simulink model "three"  (R2020b)
settings: Solver=FixedStepAuto  StartTime=0.0  StopTime=0.5  FixedStep=0.00005  RelTol=1e-3
libraries: simulink x3
settings Model: Creator=13228  LastModifiedBy=up!

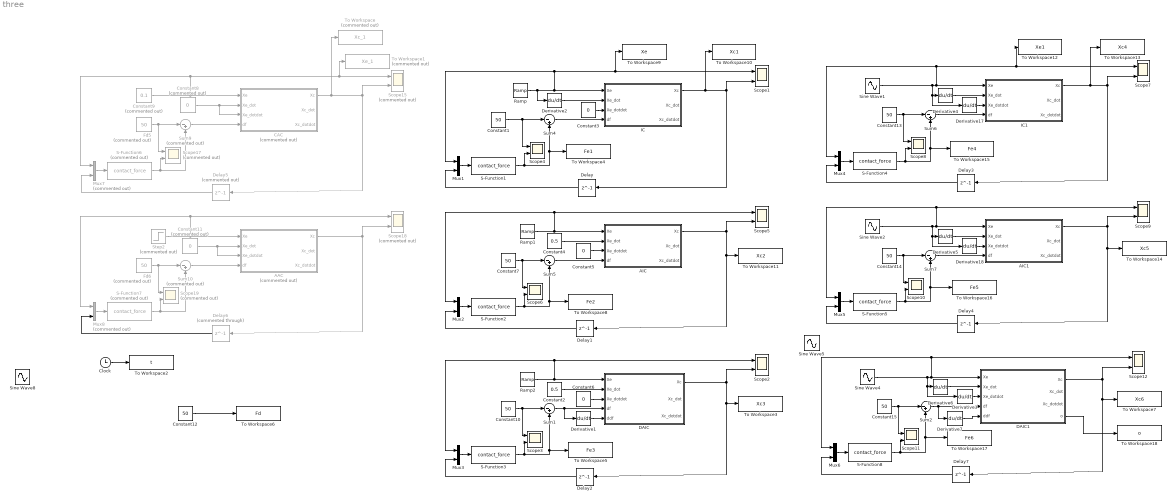
== system three ==
  AAC : MATLAB Function  Commented=on  TreatAsAtomicUnit=on
  AIC : MATLAB Function  TreatAsAtomicUnit=on
  AIC1 : MATLAB Function  TreatAsAtomicUnit=on
  CAC : MATLAB Function  Commented=on  TreatAsAtomicUnit=on
  Clock : Clock
  Constant{1,7,10,13..15} (6 alike) : Constant  Value=50
  Constant11 : Constant  Commented=on  Value=0
  Constant12 : Constant  Value=50  SampleTime=0.1
  Constant2 : Constant  Value=0.5
  Constant3 : Constant  Value=0
  Constant4 : Constant  Value=0.5
  Constant5 : Constant  Value=0
  Constant6 : Constant  Value=0
  Constant8 : Constant  Commented=on  Value=0
  Constant9 : Constant  Commented=on  Value=0.1
  DAIC : MATLAB Function  TreatAsAtomicUnit=on
  DAIC1 : MATLAB Function  TreatAsAtomicUnit=on
  Delay : Delay  DelayLength=1  InitialCondition=-0.002
  Delay1 : Delay  DelayLength=1  InitialCondition=-0.002
  Delay2 : Delay  DelayLength=1  InitialCondition=-0.002
  Delay3 : Delay  DelayLength=1  InitialCondition=0.098
  Delay4 : Delay  DelayLength=1  InitialCondition=0.098
  Delay5 : Delay  Commented=on  DelayLength=1  InitialCondition=0.098
  Delay6 : Delay  Commented=through  DelayLength=1  InitialCondition=0.098
  Delay7 : Delay  DelayLength=1  InitialCondition=0.098
  Derivative{1..7,17..18} (9 alike) : Derivative
  Fd5 : Constant  Commented=on  Value=50
  Fd6 : Constant  Commented=on  Value=50
  IC : MATLAB Function  TreatAsAtomicUnit=on
  IC1 : MATLAB Function  TreatAsAtomicUnit=on
  Mux{1..6} (6 alike) : Mux  Inputs=2
  Mux7 : Mux  Commented=on  Inputs=2
  Mux8 : Mux  Commented=on  Inputs=2
  Ramp : simulink/Sources/Ramp  slope=0.5  start=0.001  InitialOutput=0
  Ramp1 : simulink/Sources/Ramp  slope=0.5  start=0.001  InitialOutput=0
  Ramp2 : simulink/Sources/Ramp  slope=0.5  start=0.001  InitialOutput=0
  S-Function{1..5,8} (6 alike) : S-Function  FunctionName=contact_force  SFunctionDeploymentMode=off  EnableBusSupport=off
  S-Function6 : S-Function  Commented=on  FunctionName=contact_force  SFunctionDeploymentMode=off  EnableBusSupport=off
  S-Function7 : S-Function  Commented=on  FunctionName=contact_force  SFunctionDeploymentMode=off  EnableBusSupport=off
  Scope{1..12} (12 alike) : Scope  NumInputPorts=2
  Scope{15,17..19} (4 alike) : Scope  Commented=on  NumInputPorts=2
  Sine Wave1 : Sin  Amplitude=0.1  Bias=0.1  Frequency=pi  Phase=0.01  SampleTime=0
  Sine Wave2 : Sin  Amplitude=0.1  Bias=0.1  Frequency=pi  Phase=0.01  SampleTime=0
  Sine Wave4 : Sin  Amplitude=0.1  Bias=0.1  Frequency=pi  Phase=0.01  SampleTime=0
  Sine Wave5 : Sin  Amplitude=10  Bias=10  Frequency=pi  Phase=0.01  SampleTime=0
  Sine Wave8 : Sin  Amplitude=10  Bias=10  Frequency=pi  Phase=0.01  SampleTime=0
  Step2 : Step  Commented=on  Time=0  After=0.1  SampleTime=0
  Sum{1..2,4..7} (6 alike) : Sum  Inputs=|-+
  Sum10 : Sum  Commented=on  Inputs=|-+
  Sum9 : Sum  Commented=on  Inputs=|-+
  To Workspace : ToWorkspace  Commented=on  VariableName=Xc_1  SaveFormat=Timeseries  SampleTime=-1
  To Workspace1 : ToWorkspace  Commented=on  VariableName=Xe_1  SaveFormat=Timeseries  SampleTime=-1
  To Workspace10 : ToWorkspace  VariableName=Xc1  SaveFormat=Timeseries  SampleTime=-1
  To Workspace11 : ToWorkspace  VariableName=Xc2  SaveFormat=Timeseries  SampleTime=-1
  To Workspace12 : ToWorkspace  VariableName=Xe1  SaveFormat=Timeseries  SampleTime=-1
  To Workspace13 : ToWorkspace  VariableName=Xc4  SaveFormat=Timeseries  SampleTime=-1
  To Workspace14 : ToWorkspace  VariableName=Xc5  SaveFormat=Timeseries  SampleTime=-1
  To Workspace15 : ToWorkspace  VariableName=Fe4  SaveFormat=Timeseries  SampleTime=-1
  To Workspace16 : ToWorkspace  VariableName=Fe5  SaveFormat=Timeseries  SampleTime=-1
  To Workspace17 : ToWorkspace  VariableName=Fe6  SaveFormat=Timeseries  SampleTime=-1
  To Workspace18 : ToWorkspace  VariableName=o  SaveFormat=Timeseries  SampleTime=-1
  To Workspace2 : ToWorkspace  VariableName=t  SaveFormat=Timeseries  SampleTime=-1
  To Workspace3 : ToWorkspace  VariableName=Xc3  SaveFormat=Timeseries  SampleTime=-1
  To Workspace4 : ToWorkspace  VariableName=Fe1  SaveFormat=Timeseries  SampleTime=-1
  To Workspace5 : ToWorkspace  VariableName=Fe3  SaveFormat=Timeseries  SampleTime=-1
  To Workspace6 : ToWorkspace  VariableName=Fd  SaveFormat=Timeseries  SampleTime=-1
  To Workspace7 : ToWorkspace  VariableName=Xc6  SaveFormat=Timeseries  SampleTime=-1
  To Workspace8 : ToWorkspace  VariableName=Fe2  SaveFormat=Timeseries  SampleTime=-1
  To Workspace9 : ToWorkspace  VariableName=Xe  SaveFormat=Timeseries  SampleTime=-1
  wires:
  Delay5/1 -> Mux7/2
  Mux8/1 -> S-Function7/1
  Constant9/1 -> Mux7/1, To Workspace1/1, Scope15/1, CAC/1(Xe)
  Clock/1 -> To Workspace2/1
  AAC/1(Xc) -> Scope18/2, Delay6/1
  S-Function6/1 -> Scope17/2, Sum9/2
  Fd5/1 -> Scope17/1, Sum9/1
  Delay6/1 -> Mux8/2
  Constant8/1 -> CAC/3(Xe_dotdot), CAC/2(Xe_dot)
  Step2/1 -> Mux8/1, Scope18/1, AAC/1(Xe)
  Sum9/1 -> CAC/4(df)
  CAC/1(Xc) -> To Workspace/1, Scope15/2, Delay5/1
  S-Function7/1 -> Scope19/2, Sum10/2
  Mux7/1 -> S-Function6/1
  Constant11/1 -> AAC/3(Xe_dotdot), AAC/2(Xe_dot)
  Sum10/1 -> AAC/4(df)
  Fd6/1 -> Scope19/1, Sum10/1
  Mux1/1 -> S-Function1/1
  AIC/1(Xc) -> Scope5/2, To Workspace11/1, Delay1/1
  Sum5/1 -> AIC/4(df)
  IC/1(Xc) -> To Workspace10/1, Scope1/2, Delay/1
  Constant3/1 -> IC/3(Xe_dotdot)
  Constant4/1 -> AIC/2(Xe_dot)
  Constant5/1 -> AIC/3(Xe_dotdot)
  Derivative2/1 -> IC/2(Xe_dot)
  S-Function2/1 -> Scope6/2, To Workspace8/1, Sum5/2
  Constant7/1 -> Scope6/1, Sum5/1
  Delay/1 -> Mux1/2
  Sum4/1 -> IC/4(df)
  Mux2/1 -> S-Function2/1
  Ramp1/1 -> Mux2/1, Scope5/1, AIC/1(Xe)
  Constant1/1 -> Scope4/1, Sum4/1
  S-Function1/1 -> Scope4/2, To Workspace4/1, Sum4/2
  Ramp/1 -> Derivative2/1, Mux1/1, To Workspace9/1, Scope1/1, IC/1(Xe)
  Delay1/1 -> Mux2/2
  Mux3/1 -> S-Function3/1
  Ramp2/1 -> Mux3/1, Scope2/1, DAIC/1(Xe)
  Constant10/1 -> Scope3/1, Sum1/1
  S-Function3/1 -> Scope3/2, To Workspace5/1, Sum1/2
  Constant2/1 -> DAIC/2(Xe_dot)
  Sum1/1 -> Derivative1/1, DAIC/4(df)
  DAIC/1(Xc) -> Scope2/2, To Workspace3/1, Delay2/1
  Constant6/1 -> DAIC/3(Xe_dotdot)
  Delay2/1 -> Mux3/2
  Derivative1/1 -> DAIC/5(ddf)
  Sum6/1 -> IC1/4(df)
  Mux5/1 -> S-Function5/1
  Derivative17/1 -> IC1/3(Xe_dotdot)
  Sum7/1 -> AIC1/4(df)
  Mux4/1 -> S-Function4/1
  Delay4/1 -> Mux5/2
  Sine Wave2/1 -> AIC1/1(Xe), Mux5/1, Scope9/1, Derivative18/1, Derivative5/1
  AIC1/1(Xc) -> Scope9/2, To Workspace14/1, Delay4/1
  Delay3/1 -> Mux4/2
  Derivative5/1 -> AIC1/2(Xe_dot)
  Constant14/1 -> Scope10/1, Sum7/1
  IC1/1(Xc) -> To Workspace13/1, Scope7/2, Delay3/1
  Sine Wave1/1 -> Mux4/1, To Workspace12/1, Scope7/1, IC1/1(Xe), Derivative17/1, Derivative4/1
  S-Function5/1 -> Scope10/2, To Workspace16/1, Sum7/2
  S-Function4/1 -> Scope8/2, To Workspace15/1, Sum6/2
  Derivative4/1 -> IC1/2(Xe_dot)
  Derivative18/1 -> AIC1/3(Xe_dotdot)
  Constant13/1 -> Scope8/1, Sum6/1
  S-Function8/1 -> Scope11/2, To Workspace17/1, Sum2/2
  Derivative6/1 -> DAIC1/2(Xe_dot)
  DAIC1/1(Xc) -> To Workspace7/1, Delay7/1, Scope12/2
  Sine Wave4/1 -> Mux6/1, Scope12/1, DAIC1/1(Xe), Derivative3/1, Derivative6/1
  Sum2/1 -> Derivative7/1, DAIC1/4(df)
  Constant15/1 -> Scope11/1, Sum2/1
  Delay7/1 -> Mux6/2
  Mux6/1 -> S-Function8/1
  Derivative3/1 -> DAIC1/3(Xe_dotdot)
  Derivative7/1 -> DAIC1/5(ddf)
  Constant12/1 -> To Workspace6/1
  DAIC1/4(o) -> To Workspace18/1

== matlab function three/AIC ==
  settings: updateMethod=DISCRETE
  data: Xe input; Xc output; Xe_dot input; Xe_dotdot input; df input; Xc_dot output; Xc_dotdot output
function [Xc,Xc_dot,Xc_dotdot]  = fcnlmp(Xe,Xe_dot,Xe_dotdot,df)  
	m =1;b = 50;k=0;T = 0.0005;a=0.01; % 参数初始化  
	persistent Xc_pre Xc_dot_pre df_pre fi_pre;% 持久变量 https://ww2.mathworks.cn/help/matlab/ref/persistent.html  
	if isempty(Xc_pre)   
	   Xc_pre = -0.002;  
	end  
	if isempty(Xc_dot_pre)   
	   Xc_dot_pre = 0.1;  
    end  
    if isempty(df_pre)   
	   df_pre = 51;  
    end  
    if isempty(fi_pre)   
	   fi_pre = 0;  
    end  
    fi = fi_pre + a/b * df_pre;
    db = fi * b/(Xe_dot - Xc_dot_pre);
    fprintf('fi=%f,db=%f\n',fi,db);
    fi_pre = fi;
    df_pre = df;
%     db = 0;   
	Xc_dotdot_pre = Xe_dotdot + 1/m*(df + (b + db)*(Xe_dot - Xc_dot_pre) + k*(Xe - Xc_pre)); % 上一采样时间 nT 机器人末端的实际运动加速度  
	Xc = Xc_pre + Xc_dot_pre*T;           % 当前采样时间 (n+1)T 机器人末端的实际运动位置  
	Xc_dot = Xc_dot_pre + Xc_dotdot_pre*T;% 当前采样时间 (n+1)T 机器人末端的实际运动速度  
	Xc_dotdot = Xc_dotdot_pre;            % 当前采样时间 (n+1)T 机器人末端的实际运动加速度  
	Xc_dot_pre = Xc_dot;                  % 上一采样时间 nT 机器人末端的实际运动速度  
	Xc_pre = Xc;                          % 上一采样时间 nT 机器人末端的实际运动位置  
end

== matlab function three/IC ==
  settings: updateMethod=DISCRETE
  data: Xe input; Xc output; Xe_dot input; Xe_dotdot input; df input; Xc_dot output; Xc_dotdot output
function [Xc,Xc_dot,Xc_dotdot]  = fcnlmp(Xe,Xe_dot,Xe_dotdot,df)  
	m =1;b = 50;k=0;T = 0.00005; % 参数初始化  
	persistent Xc_pre Xc_dot_pre;% 持久变量 https://ww2.mathworks.cn/help/matlab/ref/persistent.html  
	if isempty(Xc_pre)   
	   Xc_pre = -0.002;  
	end  
	if isempty(Xc_dot_pre)   
	   Xc_dot_pre = 0;  
	end  
	Xc_dotdot_pre = Xe_dotdot + 1/m*(df + b*(Xe_dot - Xc_dot_pre) + k*(Xe - Xc_pre)); % 上一采样时间 nT 机器人末端的实际运动加速度  
	Xc = Xc_pre + Xc_dot_pre*T;           % 当前采样时间 (n+1)T 机器人末端的实际运动位置  
	Xc_dot = Xc_dot_pre + Xc_dotdot_pre*T;% 当前采样时间 (n+1)T 机器人末端的实际运动速度  
	Xc_dotdot = Xc_dotdot_pre;            % 当前采样时间 (n+1)T 机器人末端的实际运动加速度  
	Xc_dot_pre = Xc_dot;                  % 上一采样时间 nT 机器人末端的实际运动速度  
	Xc_pre = Xc;                          % 上一采样时间 nT 机器人末端的实际运动位置  
end

== matlab function three/DAIC ==
  settings: updateMethod=DISCRETE
  data: Xe input; Xc output; Xe_dot input; Xe_dotdot input; df input; Xc_dot output; Xc_dotdot output; ddf input
function [Xc,Xc_dot,Xc_dotdot]  = fcnlmp(Xe,Xe_dot,Xe_dotdot,df,ddf)  
	m =1;b = 50;k=0;T = 0.0005;a=2;p=0.001;U=100;e=2.7183; % 参数初始化  
	persistent Xc_pre Xc_dot_pre df_pre fi_pre;% 持久变量 https://ww2.mathworks.cn/help/matlab/ref/persistent.html  
	if isempty(Xc_pre)   
	   Xc_pre = -0.002;  
	end  
	if isempty(Xc_dot_pre)   
	   Xc_dot_pre = 0.1;  
    end  
    if isempty(df_pre)   
	   df_pre = 51;  
    end  
    if isempty(fi_pre)   
	   fi_pre = 0;  
    end  
    o=1/(e^(a/abs(df))+e^(p*abs(ddf))+U);
    fi = fi_pre + o/b * df_pre;
    db = fi * b/(Xe_dot - Xc_dot_pre);
    fprintf('fi=%f,db=%f\n',fi,db);
    fi_pre = fi;
    df_pre = df;
%     db = 0;   
	Xc_dotdot_pre = Xe_dotdot + 1/m*(df + (b + db)*(Xe_dot - Xc_dot_pre) + k*(Xe - Xc_pre)); % 上一采样时间 nT 机器人末端的实际运动加速度  
	Xc = Xc_pre + Xc_dot_pre*T;           % 当前采样时间 (n+1)T 机器人末端的实际运动位置  
	Xc_dot = Xc_dot_pre + Xc_dotdot_pre*T;% 当前采样时间 (n+1)T 机器人末端的实际运动速度  
	Xc_dotdot = Xc_dotdot_pre;            % 当前采样时间 (n+1)T 机器人末端的实际运动加速度  
	Xc_dot_pre = Xc_dot;                  % 上一采样时间 nT 机器人末端的实际运动速度  
	Xc_pre = Xc;                          % 上一采样时间 nT 机器人末端的实际运动位置  
end

== matlab function three/AIC1 ==
  settings: updateMethod=DISCRETE
  data: Xe input; Xc output; Xe_dot input; Xe_dotdot input; df input; Xc_dot output; Xc_dotdot output
function [Xc,Xc_dot,Xc_dotdot]  = fcnlmp(Xe,Xe_dot,Xe_dotdot,df)  
	m =1;b = 50;k=0;T = 0.0005;a=0.01; % 参数初始化  
	persistent Xc_pre Xc_dot_pre df_pre fi_pre;% 持久变量 https://ww2.mathworks.cn/help/matlab/ref/persistent.html  
	if isempty(Xc_pre)   
	   Xc_pre = 0.098;  
	end  
	if isempty(Xc_dot_pre)   
	   Xc_dot_pre = 0.1;  
    end  
    if isempty(df_pre)   
	   df_pre = 51;  
    end  
    if isempty(fi_pre)   
	   fi_pre = 0;  
    end  
    fi = fi_pre + a/b * df_pre;
    db = fi * b/(Xe_dot - Xc_dot_pre);
%     fprintf('fi=%f,db=%f\n',fi,db);
    fi_pre = fi;
    df_pre = df;
	Xc_dotdot_pre = Xe_dotdot + 1/m*(df + (b + db)*(Xe_dot - Xc_dot_pre) + k*(Xe - Xc_pre)); % 上一采样时间 nT 机器人末端的实际运动加速度  
	Xc = Xc_pre + Xc_dot_pre*T;           % 当前采样时间 (n+1)T 机器人末端的实际运动位置  
	Xc_dot = Xc_dot_pre + Xc_dotdot_pre*T;% 当前采样时间 (n+1)T 机器人末端的实际运动速度  
	Xc_dotdot = Xc_dotdot_pre;            % 当前采样时间 (n+1)T 机器人末端的实际运动加速度  
	Xc_dot_pre = Xc_dot;                  % 上一采样时间 nT 机器人末端的实际运动速度  
	Xc_pre = Xc;                          % 上一采样时间 nT 机器人末端的实际运动位置  
end

== matlab function three/IC1 ==
  settings: updateMethod=DISCRETE
  data: Xe input; Xc output; Xe_dot input; Xe_dotdot input; df input; Xc_dot output; Xc_dotdot output
function [Xc,Xc_dot,Xc_dotdot]  = fcnlmp(Xe,Xe_dot,Xe_dotdot,df)  
	m =1;b = 50;k=0;T = 0.00005; % 参数初始化  
	persistent Xc_pre Xc_dot_pre;% 持久变量 https://ww2.mathworks.cn/help/matlab/ref/persistent.html  
	if isempty(Xc_pre)   
	   Xc_pre = 0.098;  
	end  
	if isempty(Xc_dot_pre)   
	   Xc_dot_pre = 0;  
	end  
	Xc_dotdot_pre = Xe_dotdot + 1/m*(df + b*(Xe_dot - Xc_dot_pre) + k*(Xe - Xc_pre)); % 上一采样时间 nT 机器人末端的实际运动加速度  
	Xc = Xc_pre + Xc_dot_pre*T;           % 当前采样时间 (n+1)T 机器人末端的实际运动位置  
	Xc_dot = Xc_dot_pre + Xc_dotdot_pre*T;% 当前采样时间 (n+1)T 机器人末端的实际运动速度  
	Xc_dotdot = Xc_dotdot_pre;            % 当前采样时间 (n+1)T 机器人末端的实际运动加速度  
	Xc_dot_pre = Xc_dot;                  % 上一采样时间 nT 机器人末端的实际运动速度  
	Xc_pre = Xc;                          % 上一采样时间 nT 机器人末端的实际运动位置  
end

== matlab function three/CAC ==
  settings: updateMethod=DISCRETE
  data: Xe input; Xc output; Xe_dot input; Xe_dotdot input; df input; Xc_dot output; Xc_dotdot output
function [Xc,Xc_dot,Xc_dotdot]  = fcnlmp(Xe,Xe_dot,Xe_dotdot,df)  
	m =1;b = 60;k=0;T = 0.00005; % 参数初始化  
	persistent Xc_pre Xc_dot_pre;% 持久变量 https://ww2.mathworks.cn/help/matlab/ref/persistent.html  
	if isempty(Xc_pre)   
	   Xc_pre = 0.098;  
	end  
	if isempty(Xc_dot_pre)   
	   Xc_dot_pre = 0;  
	end  
	Xc_dotdot_pre = Xe_dotdot + 1/m*(df + b*(Xe_dot - Xc_dot_pre) + k*(Xe - Xc_pre)); % 上一采样时间 nT 机器人末端的实际运动加速度  
	Xc = Xc_pre + Xc_dot_pre*T;           % 当前采样时间 (n+1)T 机器人末端的实际运动位置  
	Xc_dot = Xc_dot_pre + Xc_dotdot_pre*T;% 当前采样时间 (n+1)T 机器人末端的实际运动速度  
	Xc_dotdot = Xc_dotdot_pre;            % 当前采样时间 (n+1)T 机器人末端的实际运动加速度  
	Xc_dot_pre = Xc_dot;                  % 上一采样时间 nT 机器人末端的实际运动速度  
	Xc_pre = Xc;                          % 上一采样时间 nT 机器人末端的实际运动位置  
end

== matlab function three/AAC ==
  settings: updateMethod=DISCRETE
  data: Xe input; Xc output; Xe_dot input; Xe_dotdot input; df input; Xc_dot output; Xc_dotdot output
function [Xc,Xc_dot,Xc_dotdot]  = fcnlmp(Xe,Xe_dot,Xe_dotdot,df)  
	m =1;b = 100;k=0;T = 0.005;a=0.01; % 参数初始化  
	persistent Xc_pre Xc_dot_pre df_pre fi_pre;% 持久变量 https://ww2.mathworks.cn/help/matlab/ref/persistent.html  
	if isempty(Xc_pre)   
	   Xc_pre = 0.098;  
	end  
	if isempty(Xc_dot_pre)   
	   Xc_dot_pre = 0.1;  
    end  
    if isempty(df_pre)   
	   df_pre = 51;  
    end  
    if isempty(fi_pre)   
	   fi_pre = 0;  
    end  
    fi = fi_pre + a/b * df_pre;
    db = fi * b/(Xe_dot - Xc_dot_pre);
    fprintf('fi=%f,db=%f\n',fi,db);
    fi_pre = fi;
    df_pre = df;
%     db = 0;   
	Xc_dotdot_pre = Xe_dotdot + 1/m*(df + (b + db)*(Xe_dot - Xc_dot_pre) + k*(Xe - Xc_pre)); % 上一采样时间 nT 机器人末端的实际运动加速度  
	Xc = Xc_pre + Xc_dot_pre*T;           % 当前采样时间 (n+1)T 机器人末端的实际运动位置  
	Xc_dot = Xc_dot_pre + Xc_dotdot_pre*T;% 当前采样时间 (n+1)T 机器人末端的实际运动速度  
	Xc_dotdot = Xc_dotdot_pre;            % 当前采样时间 (n+1)T 机器人末端的实际运动加速度  
	Xc_dot_pre = Xc_dot;                  % 上一采样时间 nT 机器人末端的实际运动速度  
	Xc_pre = Xc;                          % 上一采样时间 nT 机器人末端的实际运动位置  
end

== matlab function three/DAIC1 ==
  settings: updateMethod=DISCRETE
  data: Xe input; Xc output; Xe_dot input; Xe_dotdot input; df input; Xc_dot output; Xc_dotdot output; ddf input; o output
function [Xc,Xc_dot,Xc_dotdot,o]  = fcnlmp(Xe,Xe_dot,Xe_dotdot,df,ddf)  
	m =1;b = 50;k=0;T = 0.0005;a=2;p=0.001;U=100;e=2.7183; % 参数初始化  
	persistent Xc_pre Xc_dot_pre df_pre fi_pre;% 持久变量 https://ww2.mathworks.cn/help/matlab/ref/persistent.html  
	if isempty(Xc_pre)   
	   Xc_pre = 0.098;  
	end  
	if isempty(Xc_dot_pre)   
	   Xc_dot_pre = 0.1;  
    end  
    if isempty(df_pre)   
	   df_pre = 51;  
    end  
    if isempty(fi_pre)   
	   fi_pre = 0;  
    end  
    o=1/(e^(a/abs(df))+e^(p*abs(ddf))+U);
    fi = fi_pre + o/b * df_pre;
    db = fi * b/(Xe_dot - Xc_dot_pre);
    fprintf('fi=%f,db=%f\n',fi,db);
    fi_pre = fi;
    df_pre = df;
%     db = 0;   
	Xc_dotdot_pre = Xe_dotdot + 1/m*(df + (b + db)*(Xe_dot - Xc_dot_pre) + k*(Xe - Xc_pre)); % 上一采样时间 nT 机器人末端的实际运动加速度  
	Xc = Xc_pre + Xc_dot_pre*T;           % 当前采样时间 (n+1)T 机器人末端的实际运动位置  
	Xc_dot = Xc_dot_pre + Xc_dotdot_pre*T;% 当前采样时间 (n+1)T 机器人末端的实际运动速度  
	Xc_dotdot = Xc_dotdot_pre;            % 当前采样时间 (n+1)T 机器人末端的实际运动加速度  
	Xc_dot_pre = Xc_dot;                  % 上一采样时间 nT 机器人末端的实际运动速度  
	Xc_pre = Xc;                          % 上一采样时间 nT 机器人末端的实际运动位置  
end
